simulink model "NMM_order6_multi2"  (R2023a)
settings: Solver=VariableStepAuto  StartTime=0.0  StopTime=11.0  RelTol=1e-3
undefined symbols (not defined in the file): clf
libraries: simulink x4
(part 1 of 2)
settings Model: Creator=HP  LastModifiedBy=admin

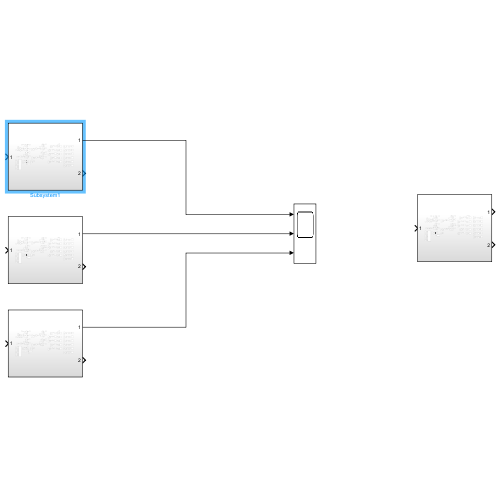
[thumbnail: Simulink's stored preview of the top-level diagram]
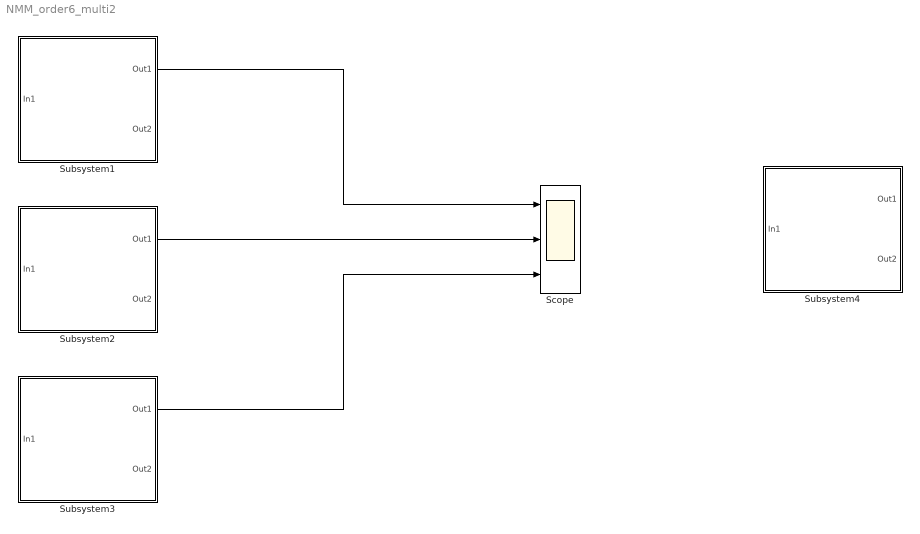
== system NMM_order6_multi2 ==
  Scope : Scope  NumInputPorts=3
  Subsystem1 : Subsystem
  Subsystem2 : Subsystem
  Subsystem3 : Subsystem
  Subsystem4 : Subsystem
  wires:
  Subsystem1/1(Out1) -> Scope/1
  Subsystem2/1(Out1) -> Scope/2
  Subsystem3/1(Out1) -> Scope/3

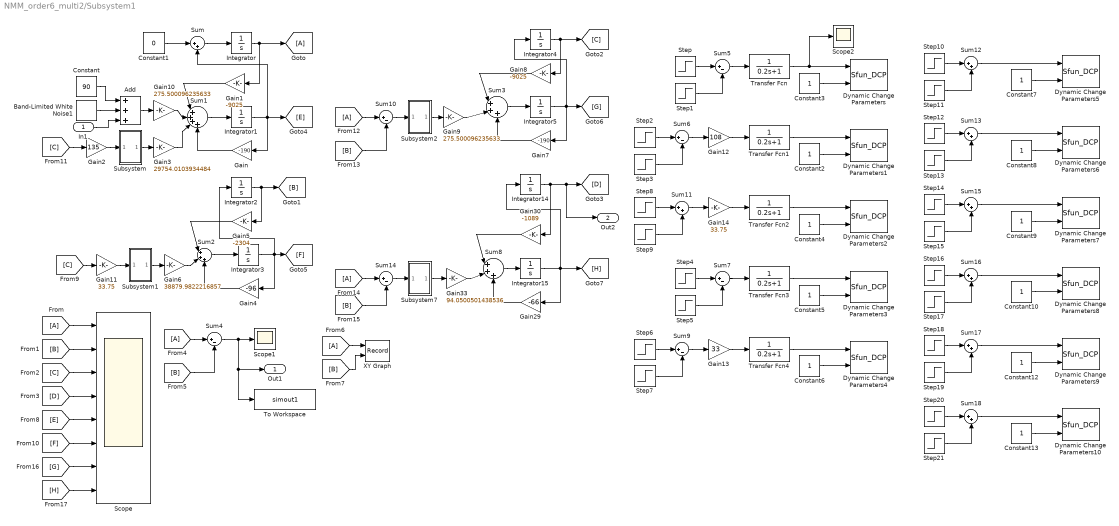
== system NMM_order6_multi2/Subsystem1 ==
  In1 : Inport
  Add : Sum  Inputs=+++
  Band-Limited White Noise1 : simulink/Sources/Band-Limited White Noise  Cov=[0.03]  Ts=0.001  seed=[23341]
  Constant : Constant  Value=90
  Constant1 : Constant  Value=0
  Constant{2..10,12..13} (11 alike) : Constant
  Dynamic Change Parameters : M-S-Function  StopFcn=close(clf)  FunctionName=Sfun_DCP  Parameters=block_name,par_name,sample_time,dimension  mask{block_name='NMM_order6_multi2/Subsystem1/Gain10', par_name='Gain', reset=off, sample_time=[0.01 0], dimension=[1 1]}
      mask help:
      | Dynamic Change Parameters : Change Block's Parameter When the Model is running
      |
      | block_name : name of the block  need to change parameter,must be string
      | par_name   : name of the parameter want to change,must be string
      | sample_time: sample time of this block
      | demension  : demension of the parameter want to change,must be [m n]
      mask Callback reset:
      | if strcmp( get_param(gcb,'reset'),'on' )
      |    fig_par_set();
      | end
      mask Callback sample_time:
      | st = get_param(gcb,'sample_time');
      | st = str2num(st);
      | if length(st)~=2
      |     msgbox('Sample Time is invalid ');
      | end
      mask Callback dimension:
      | st = get_param(gcb,'dimension');
      | st = str2num(st);
      | if length(st)~=2
      |     msgbox('Fromat of Dimension must be [m n]');
      | end
  Dynamic Change Parameters1 : M-S-Function  StopFcn=close(clf)  FunctionName=Sfun_DCP  Parameters=block_name,par_name,sample_time,dimension  mask{block_name='NMM_order6_multi2/Subsystem1/Gain3', par_name='Gain', reset=off, sample_time=[0.01 0], dimension=[1 1]}
      mask help:
      | Dynamic Change Parameters : Change Block's Parameter When the Model is running
      |
      | block_name : name of the block  need to change parameter,must be string
      | par_name   : name of the parameter want to change,must be string
      | sample_time: sample time of this block
      | demension  : demension of the parameter want to change,must be [m n]
      mask Callback reset:
      | if strcmp( get_param(gcb,'reset'),'on' )
      |    fig_par_set();
      | end
      mask Callback sample_time:
      | st = get_param(gcb,'sample_time');
      | st = str2num(st);
      | if length(st)~=2
      |     msgbox('Sample Time is invalid ');
      | end
      mask Callback dimension:
      | st = get_param(gcb,'dimension');
      | st = str2num(st);
      | if length(st)~=2
      |     msgbox('Fromat of Dimension must be [m n]');
      | end
  Dynamic Change Parameters10 : M-S-Function  StopFcn=close(clf)  FunctionName=Sfun_DCP  Parameters=block_name,par_name,sample_time,dimension  mask{block_name='NMM_order6_multi2/Subsystem1/Gain7', par_name='Gain', reset=off, sample_time=[0.01 0], dimension=[1 1]}
      mask help:
      | Dynamic Change Parameters : Change Block's Parameter When the Model is running
      |
      | block_name : name of the block  need to change parameter,must be string
      | par_name   : name of the parameter want to change,must be string
      | sample_time: sample time of this block
      | demension  : demension of the parameter want to change,must be [m n]
      mask Callback reset:
      | if strcmp( get_param(gcb,'reset'),'on' )
      |    fig_par_set();
      | end
      mask Callback sample_time:
      | st = get_param(gcb,'sample_time');
      | st = str2num(st);
      | if length(st)~=2
      |     msgbox('Sample Time is invalid ');
      | end
      mask Callback dimension:
      | st = get_param(gcb,'dimension');
      | st = str2num(st);
      | if length(st)~=2
      |     msgbox('Fromat of Dimension must be [m n]');
      | end
  Dynamic Change Parameters2 : M-S-Function  StopFcn=close(clf)  FunctionName=Sfun_DCP  Parameters=block_name,par_name,sample_time,dimension  mask{block_name='NMM_order6_multi2/Subsystem1/Gain6', par_name='Gain', reset=off, sample_time=[0.01 0], dimension=[1 1]}
      mask help:
      | Dynamic Change Parameters : Change Block's Parameter When the Model is running
      |
      | block_name : name of the block  need to change parameter,must be string
      | par_name   : name of the parameter want to change,must be string
      | sample_time: sample time of this block
      | demension  : demension of the parameter want to change,must be [m n]
      mask Callback reset:
      | if strcmp( get_param(gcb,'reset'),'on' )
      |    fig_par_set();
      | end
      mask Callback sample_time:
      | st = get_param(gcb,'sample_time');
      | st = str2num(st);
      | if length(st)~=2
      |     msgbox('Sample Time is invalid ');
      | end
      mask Callback dimension:
      | st = get_param(gcb,'dimension');
      | st = str2num(st);
      | if length(st)~=2
      |     msgbox('Fromat of Dimension must be [m n]');
      | end
  Dynamic Change Parameters3 : M-S-Function  StopFcn=close(clf)  FunctionName=Sfun_DCP  Parameters=block_name,par_name,sample_time,dimension  mask{block_name='NMM_order6_multi2/Subsystem1/Gain9', par_name='Gain', reset=off, sample_time=[0.01 0], dimension=[1 1]}
      mask help:
      | Dynamic Change Parameters : Change Block's Parameter When the Model is running
      |
      | block_name : name of the block  need to change parameter,must be string
      | par_name   : name of the parameter want to change,must be string
      | sample_time: sample time of this block
      | demension  : demension of the parameter want to change,must be [m n]
      mask Callback reset:
      | if strcmp( get_param(gcb,'reset'),'on' )
      |    fig_par_set();
      | end
      mask Callback sample_time:
      | st = get_param(gcb,'sample_time');
      | st = str2num(st);
      | if length(st)~=2
      |     msgbox('Sample Time is invalid ');
      | end
      mask Callback dimension:
      | st = get_param(gcb,'dimension');
      | st = str2num(st);
      | if length(st)~=2
      |     msgbox('Fromat of Dimension must be [m n]');
      | end
  Dynamic Change Parameters4 : M-S-Function  StopFcn=close(clf)  FunctionName=Sfun_DCP  Parameters=block_name,par_name,sample_time,dimension  mask{block_name='NMM_order6_multi2/Subsystem1/Gain33', par_name='Gain', reset=off, sample_time=[0.01 0], dimension=[1 1]}
      mask help:
      | Dynamic Change Parameters : Change Block's Parameter When the Model is running
      |
      | block_name : name of the block  need to change parameter,must be string
      | par_name   : name of the parameter want to change,must be string
      | sample_time: sample time of this block
      | demension  : demension of the parameter want to change,must be [m n]
      mask Callback reset:
      | if strcmp( get_param(gcb,'reset'),'on' )
      |    fig_par_set();
      | end
      mask Callback sample_time:
      | st = get_param(gcb,'sample_time');
      | st = str2num(st);
      | if length(st)~=2
      |     msgbox('Sample Time is invalid ');
      | end
      mask Callback dimension:
      | st = get_param(gcb,'dimension');
      | st = str2num(st);
      | if length(st)~=2
      |     msgbox('Fromat of Dimension must be [m n]');
      | end
  Dynamic Change Parameters5 : M-S-Function  StopFcn=close(clf)  FunctionName=Sfun_DCP  Parameters=block_name,par_name,sample_time,dimension  mask{block_name='NMM_order6_multi2/Subsystem1/Gain1', par_name='Gain', reset=off, sample_time=[0.01 0], dimension=[1 1]}
      mask help:
      | Dynamic Change Parameters : Change Block's Parameter When the Model is running
      |
      | block_name : name of the block  need to change parameter,must be string
      | par_name   : name of the parameter want to change,must be string
      | sample_time: sample time of this block
      | demension  : demension of the parameter want to change,must be [m n]
      mask Callback reset:
      | if strcmp( get_param(gcb,'reset'),'on' )
      |    fig_par_set();
      | end
      mask Callback sample_time:
      | st = get_param(gcb,'sample_time');
      | st = str2num(st);
      | if length(st)~=2
      |     msgbox('Sample Time is invalid ');
      | end
      mask Callback dimension:
      | st = get_param(gcb,'dimension');
      | st = str2num(st);
      | if length(st)~=2
      |     msgbox('Fromat of Dimension must be [m n]');
      | end
  Dynamic Change Parameters6 : M-S-Function  StopFcn=close(clf)  FunctionName=Sfun_DCP  Parameters=block_name,par_name,sample_time,dimension  mask{block_name='NMM_order6_multi2/Subsystem1/Gain', par_name='Gain', reset=off, sample_time=[0.01 0], dimension=[1 1]}
      mask help:
      | Dynamic Change Parameters : Change Block's Parameter When the Model is running
      |
      | block_name : name of the block  need to change parameter,must be string
      | par_name   : name of the parameter want to change,must be string
      | sample_time: sample time of this block
      | demension  : demension of the parameter want to change,must be [m n]
      mask Callback reset:
      | if strcmp( get_param(gcb,'reset'),'on' )
      |    fig_par_set();
      | end
      mask Callback sample_time:
      | st = get_param(gcb,'sample_time');
      | st = str2num(st);
      | if length(st)~=2
      |     msgbox('Sample Time is invalid ');
      | end
      mask Callback dimension:
      | st = get_param(gcb,'dimension');
      | st = str2num(st);
      | if length(st)~=2
      |     msgbox('Fromat of Dimension must be [m n]');
      | end
  Dynamic Change Parameters7 : M-S-Function  StopFcn=close(clf)  FunctionName=Sfun_DCP  Parameters=block_name,par_name,sample_time,dimension  mask{block_name='NMM_order6_multi2/Subsystem1/Gain5', par_name='Gain', reset=off, sample_time=[0.01 0], dimension=[1 1]}
      mask help:
      | Dynamic Change Parameters : Change Block's Parameter When the Model is running
      |
      | block_name : name of the block  need to change parameter,must be string
      | par_name   : name of the parameter want to change,must be string
      | sample_time: sample time of this block
      | demension  : demension of the parameter want to change,must be [m n]
      mask Callback reset:
      | if strcmp( get_param(gcb,'reset'),'on' )
      |    fig_par_set();
      | end
      mask Callback sample_time:
      | st = get_param(gcb,'sample_time');
      | st = str2num(st);
      | if length(st)~=2
      |     msgbox('Sample Time is invalid ');
      | end
      mask Callback dimension:
      | st = get_param(gcb,'dimension');
      | st = str2num(st);
      | if length(st)~=2
      |     msgbox('Fromat of Dimension must be [m n]');
      | end
  Dynamic Change Parameters8 : M-S-Function  StopFcn=close(clf)  FunctionName=Sfun_DCP  Parameters=block_name,par_name,sample_time,dimension  mask{block_name='NMM_order6_multi2/Subsystem1/Gain4', par_name='Gain', reset=off, sample_time=[0.01 0], dimension=[1 1]}
      mask help:
      | Dynamic Change Parameters : Change Block's Parameter When the Model is running
      |
      | block_name : name of the block  need to change parameter,must be string
      | par_name   : name of the parameter want to change,must be string
      | sample_time: sample time of this block
      | demension  : demension of the parameter want to change,must be [m n]
      mask Callback reset:
      | if strcmp( get_param(gcb,'reset'),'on' )
      |    fig_par_set();
      | end
      mask Callback sample_time:
      | st = get_param(gcb,'sample_time');
      | st = str2num(st);
      | if length(st)~=2
      |     msgbox('Sample Time is invalid ');
      | end
      mask Callback dimension:
      | st = get_param(gcb,'dimension');
      | st = str2num(st);
      | if length(st)~=2
      |     msgbox('Fromat of Dimension must be [m n]');
      | end
  Dynamic Change Parameters9 : M-S-Function  StopFcn=close(clf)  FunctionName=Sfun_DCP  Parameters=block_name,par_name,sample_time,dimension  mask{block_name='NMM_order6_multi2/Subsystem1/Gain8', par_name='Gain', reset=off, sample_time=[0.01 0], dimension=[1 1]}
      mask help:
      | Dynamic Change Parameters : Change Block's Parameter When the Model is running
      |
      | block_name : name of the block  need to change parameter,must be string
      | par_name   : name of the parameter want to change,must be string
      | sample_time: sample time of this block
      | demension  : demension of the parameter want to change,must be [m n]
      mask Callback reset:
      | if strcmp( get_param(gcb,'reset'),'on' )
      |    fig_par_set();
      | end
      mask Callback sample_time:
      | st = get_param(gcb,'sample_time');
      | st = str2num(st);
      | if length(st)~=2
      |     msgbox('Sample Time is invalid ');
      | end
      mask Callback dimension:
      | st = get_param(gcb,'dimension');
      | st = str2num(st);
      | if length(st)~=2
      |     msgbox('Fromat of Dimension must be [m n]');
      | end
  From{,4,6,12,14} (5 alike) : From
  Gain : Gain  Gain=-190
  Gain1 : Gain  Gain=-9025
  Gain10 : Gain  Gain=275.500096235633
  Gain11 : Gain  Gain=33.75
  Gain12 : Gain  Gain=108
  Gain13 : Gain  Gain=33
  Gain14 : Gain  Gain=33.75
  Gain2 : Gain  Gain=135
  Gain29 : Gain  Gain=-66
  Gain3 : Gain  Gain=29754.0103934484
  Gain30 : Gain  Gain=-1089
  Gain33 : Gain  Gain=94.0500501438536
  Gain4 : Gain  Gain=-96
  Gain5 : Gain  Gain=-2304
  Gain6 : Gain  Gain=38879.9822216857
  Gain7 : Gain  Gain=-190
  Gain8 : Gain  Gain=-9025
  Gain9 : Gain  Gain=275.500096235633
  Goto : Goto
  Integrator{,1..5,14..15} (8 alike) : Integrator
  Scope : Scope  NumInputPorts=8
  Scope1 : Scope
  Scope2 : Scope
  Step : Step  Time=5.8  Before=2.35*100  After=3.00*95  SampleTime=0
  Step1 : Step  Time=8.7  After=9.5  SampleTime=0
  Step10 : Step  Time=5.8  Before=-10000  After=-9025  SampleTime=0
  Step{11,13,15,17,19,21} (6 alike) : Step  Time=8.7  After=0  SampleTime=0
  Step12 : Step  Time=5.8  Before=-200  After=-190  SampleTime=0
  Step14 : Step  Time=5.8  Before=-2500  After=-2304  SampleTime=0
  Step16 : Step  Time=5.8  Before=-100  After=-96  SampleTime=0
  Step18 : Step  Time=5.8  Before=-10000  After=-9025  SampleTime=0
  Step2 : Step  Time=5.8  Before=2.35*100  After=3.00*95  SampleTime=0
  Step20 : Step  Time=5.8  Before=-200  After=-190  SampleTime=0
  Step3 : Step  Time=8.7  After=9.5  SampleTime=0
  Step4 : Step  Time=5.8  Before=2.35*100  After=3.00*95  SampleTime=0
  Step5 : Step  Time=8.7  After=9.5  SampleTime=0
  Step6 : Step  Time=5.8  Before=2.35  After=3.00  SampleTime=0
  Step7 : Step  Time=8.7  After=0.15  SampleTime=0
  Step8 : Step  Time=20  Before=22*50  After=22*50  SampleTime=0
  Step9 : Step  Time=8.7  After=52  SampleTime=0
  Subsystem : Subsystem
  Subsystem1 : Subsystem
  Subsystem2 : Subsystem
  Subsystem7 : Subsystem
  Sum{,11..13,15..18} (8 alike) : Sum  Inputs=|++
  Sum1 : Sum  Inputs=|++++
  Sum{4..7,9..10,14} (7 alike) : Sum  Inputs=|+-
  Sum2 : Sum  Inputs=|+++
  Sum3 : Sum  Inputs=|+++
  Sum8 : Sum  Inputs=|+++
  To Workspace : ToWorkspace  VariableName=simout1  SaveFormat=Timeseries  SampleTime=-1
  Transfer Fcn{,1..4} (5 alike) : TransferFcn  Denominator=[0.2 1]
  XY Graph : Record  FileSettingsInternal="{\"entries\":[{\"content\":{\"excelSettings\":{\"content\":{},\"type\":\"Streamout.ExcelSettings\"}},\"type\":\"Streamout.FileSettingStorage\",\"uuid\":\"\"}],\"packageUris\":[\"http:\\/\\/schema.mathworks.com\\/mf0\\/streamout_blocks\\/R2020a\"],\"version\":\"1.0\"}"  Layout=[1 1]  SignalsInternal="{\"entries\":[{\"content\":{\"signals\":[{\"content\":{\"blockPath\":[],\"dimensions\":[1],\"domain\":\"\",\"lineColor\":\"#77ac30\",\"port\":1,\"sid\":[\"\"],\"signalID\":93784,\"signalName\":\"From6\"},\"type\":\"RecordBlkView.Signal\",\"uuid\":\"\"},{\"content\":{\"blockPath\":[],\"dimensions\":[1],\"domain\":\"\",\"lineColor\":\"#4dbeee\",\"port\":2,\"sid\":[\"\"],\"signalID\":93788,\"signalName\":\"From7\"},\"type\":\"RecordBlkView.Signal\",\"uuid\":\"\"}]},\"type\":\"RecordBlkView.InputSignals\",\"uuid\":\"\"}],\"packageUris\":[\"http:\\/\\/schema.mathworks.com\\/mf0\\/streamout_blocks\\/R2020a\"],\"version\":\"1.0\"}"  VisualizationBindings="{\"xyplotplugin\":{\"info\":[{\"series\":[],\"subplotID\":1}]}}"  CompatibilityTag=XY
  Out1 : Outport
  Out2 : Outport  Port=2
  wires:
  Sum4/1 -> To Workspace/1, Out1/1, Scope1/1
  [C] -> Scope/3
  Gain1/1 -> Sum1/1
  Sum1/1 -> Integrator1/1
  Subsystem2/1(Out2) -> Gain9/1
  [B] -> Sum10/2
  [G] -> Scope/7
  Subsystem/1(Out2) -> Gain3/1
  Gain4/1 -> Sum2/3
  Gain9/1 -> Sum3/2
  [D] -> Scope/4
  Integrator4/1 -> [C], Gain8/1
  Sum/1 -> Integrator/1
  Gain3/1 -> Sum1/3
  Gain30/1 -> Sum8/1
  From/1 -> Scope/1
  Constant/1 -> Add/1
  [B] -> Scope/2
  From6/1 -> XY Graph/1
  Add/1 -> Gain10/1
  Integrator5/1 -> [G], Gain7/1, Integrator4/1
  Gain/1 -> Sum1/4
  Integrator2/1 -> [B], Gain5/1
  [H] -> Scope/8
  [B] -> Sum14/2
  Integrator1/1 -> [E], Sum/2, Gain/1
  Integrator/1 -> Goto/1, Gain1/1
  Gain6/1 -> Sum2/2
  Sum8/1 -> Integrator15/1
  Integrator3/1 -> [F], Gain4/1, Integrator2/1
  Gain5/1 -> Sum2/1
  Gain8/1 -> Sum3/1
  Integrator14/1 -> Out2/1, [D], Gain30/1
  Integrator15/1 -> [H], Gain29/1, Integrator14/1
  Subsystem1/1(Out2) -> Gain6/1
  From14/1 -> Sum14/1
  Gain2/1 -> Subsystem/1(In1)
  Sum14/1 -> Subsystem7/1(In1)
  Sum10/1 -> Subsystem2/1(In1)
  Gain33/1 -> Sum8/2
  Gain29/1 -> Sum8/3
  [C] -> Gain11/1
  Subsystem7/1(Out2) -> Gain33/1
  Gain7/1 -> Sum3/3
  [B] -> Sum4/2
  From4/1 -> Sum4/1
  Band-Limited White Noise1/1 -> Add/2
  In1/1 -> Add/3
  Sum3/1 -> Integrator5/1
  Constant1/1 -> Sum/1
  Gain11/1 -> Subsystem1/1(In1)
  [E] -> Scope/5
  [C] -> Gain2/1
  Sum2/1 -> Integrator3/1
  [F] -> Scope/6
  Gain10/1 -> Sum1/2
  From12/1 -> Sum10/1
  [B] -> XY Graph/2
  Constant3/1 -> Dynamic Change Parameters/2
  Constant2/1 -> Dynamic Change Parameters1/2
  Constant5/1 -> Dynamic Change Parameters3/2
  Constant6/1 -> Dynamic Change Parameters4/2
  Step/1 -> Sum5/1
  Step1/1 -> Sum5/2
  Step3/1 -> Sum6/2
  Step2/1 -> Sum6/1
  Sum6/1 -> Gain12/1
  Step5/1 -> Sum7/2
  Step4/1 -> Sum7/1
  Step7/1 -> Sum9/2
  Step6/1 -> Sum9/1
  Sum9/1 -> Gain13/1
  Step9/1 -> Sum11/2
  Step8/1 -> Sum11/1
  Sum11/1 -> Gain14/1
  Constant4/1 -> Dynamic Change Parameters2/2
  Sum5/1 -> Transfer Fcn/1
  Transfer Fcn/1 -> Scope2/1, Dynamic Change Parameters/1
  Transfer Fcn1/1 -> Dynamic Change Parameters1/1
  Gain12/1 -> Transfer Fcn1/1
  Gain14/1 -> Transfer Fcn2/1
  Transfer Fcn2/1 -> Dynamic Change Parameters2/1
  Sum7/1 -> Transfer Fcn3/1
  Transfer Fcn3/1 -> Dynamic Change Parameters3/1
  Gain13/1 -> Transfer Fcn4/1
  Transfer Fcn4/1 -> Dynamic Change Parameters4/1
  Step11/1 -> Sum12/2
  Constant7/1 -> Dynamic Change Parameters5/2
  Step10/1 -> Sum12/1
  Step13/1 -> Sum13/2
  Constant8/1 -> Dynamic Change Parameters6/2
  Step12/1 -> Sum13/1
  Step16/1 -> Sum16/1
  Constant10/1 -> Dynamic Change Parameters8/2
  Step17/1 -> Sum16/2
  Constant9/1 -> Dynamic Change Parameters7/2
  Step15/1 -> Sum15/2
  Step14/1 -> Sum15/1
  Constant13/1 -> Dynamic Change Parameters10/2
  Step21/1 -> Sum18/2
  Step19/1 -> Sum17/2
  Constant12/1 -> Dynamic Change Parameters9/2
  Step20/1 -> Sum18/1
  Step18/1 -> Sum17/1
  Sum12/1 -> Dynamic Change Parameters5/1
  Sum13/1 -> Dynamic Change Parameters6/1
  Sum15/1 -> Dynamic Change Parameters7/1
  Sum16/1 -> Dynamic Change Parameters8/1
  Sum17/1 -> Dynamic Change Parameters9/1
  Sum18/1 -> Dynamic Change Parameters10/1

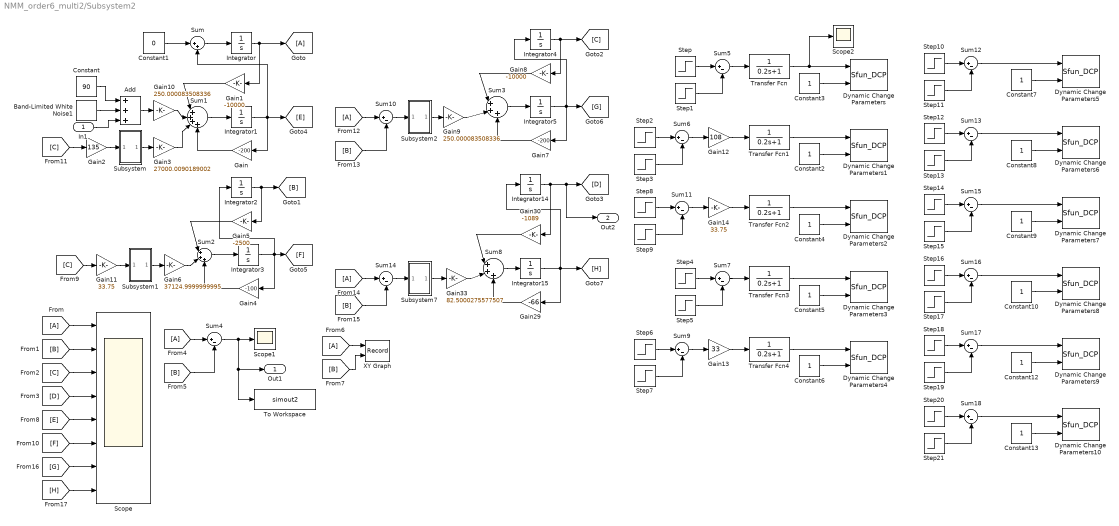
== system NMM_order6_multi2/Subsystem2 ==
  In1 : Inport
  Add : Sum  Inputs=+++
  Band-Limited White Noise1 : simulink/Sources/Band-Limited White Noise  Cov=[0.01]  Ts=0.001  seed=[35471]
  Constant : Constant  Value=90
  Constant1 : Constant  Value=0
  Constant{2..10,12..13} (11 alike) : Constant
  Dynamic Change Parameters : M-S-Function  StopFcn=close(clf)  FunctionName=Sfun_DCP  Parameters=block_name,par_name,sample_time,dimension  mask{block_name='NMM_order6_multi2/Subsystem2/Gain10', par_name='Gain', reset=off, sample_time=[0.01 0], dimension=[1 1]}
      mask help:
      | Dynamic Change Parameters : Change Block's Parameter When the Model is running
      |
      | block_name : name of the block  need to change parameter,must be string
      | par_name   : name of the parameter want to change,must be string
      | sample_time: sample time of this block
      | demension  : demension of the parameter want to change,must be [m n]
      mask Callback reset:
      | if strcmp( get_param(gcb,'reset'),'on' )
      |    fig_par_set();
      | end
      mask Callback sample_time:
      | st = get_param(gcb,'sample_time');
      | st = str2num(st);
      | if length(st)~=2
      |     msgbox('Sample Time is invalid ');
      | end
      mask Callback dimension:
      | st = get_param(gcb,'dimension');
      | st = str2num(st);
      | if length(st)~=2
      |     msgbox('Fromat of Dimension must be [m n]');
      | end
  Dynamic Change Parameters1 : M-S-Function  StopFcn=close(clf)  FunctionName=Sfun_DCP  Parameters=block_name,par_name,sample_time,dimension  mask{block_name='NMM_order6_multi2/Subsystem2/Gain3', par_name='Gain', reset=off, sample_time=[0.01 0], dimension=[1 1]}
      mask help:
      | Dynamic Change Parameters : Change Block's Parameter When the Model is running
      |
      | block_name : name of the block  need to change parameter,must be string
      | par_name   : name of the parameter want to change,must be string
      | sample_time: sample time of this block
      | demension  : demension of the parameter want to change,must be [m n]
      mask Callback reset:
      | if strcmp( get_param(gcb,'reset'),'on' )
      |    fig_par_set();
      | end
      mask Callback sample_time:
      | st = get_param(gcb,'sample_time');
      | st = str2num(st);
      | if length(st)~=2
      |     msgbox('Sample Time is invalid ');
      | end
      mask Callback dimension:
      | st = get_param(gcb,'dimension');
      | st = str2num(st);
      | if length(st)~=2
      |     msgbox('Fromat of Dimension must be [m n]');
      | end
  Dynamic Change Parameters10 : M-S-Function  StopFcn=close(clf)  FunctionName=Sfun_DCP  Parameters=block_name,par_name,sample_time,dimension  mask{block_name='NMM_order6_multi2/Subsystem2/Gain7', par_name='Gain', reset=off, sample_time=[0.01 0], dimension=[1 1]}
      mask help:
      | Dynamic Change Parameters : Change Block's Parameter When the Model is running
      |
      | block_name : name of the block  need to change parameter,must be string
      | par_name   : name of the parameter want to change,must be string
      | sample_time: sample time of this block
      | demension  : demension of the parameter want to change,must be [m n]
      mask Callback reset:
      | if strcmp( get_param(gcb,'reset'),'on' )
      |    fig_par_set();
      | end
      mask Callback sample_time:
      | st = get_param(gcb,'sample_time');
      | st = str2num(st);
      | if length(st)~=2
      |     msgbox('Sample Time is invalid ');
      | end
      mask Callback dimension:
      | st = get_param(gcb,'dimension');
      | st = str2num(st);
      | if length(st)~=2
      |     msgbox('Fromat of Dimension must be [m n]');
      | end
  Dynamic Change Parameters2 : M-S-Function  StopFcn=close(clf)  FunctionName=Sfun_DCP  Parameters=block_name,par_name,sample_time,dimension  mask{block_name='NMM_order6_multi2/Subsystem2/Gain6', par_name='Gain', reset=off, sample_time=[0.01 0], dimension=[1 1]}
      mask help:
      | Dynamic Change Parameters : Change Block's Parameter When the Model is running
      |
      | block_name : name of the block  need to change parameter,must be string
      | par_name   : name of the parameter want to change,must be string
      | sample_time: sample time of this block
      | demension  : demension of the parameter want to change,must be [m n]
      mask Callback reset:
      | if strcmp( get_param(gcb,'reset'),'on' )
      |    fig_par_set();
      | end
      mask Callback sample_time:
      | st = get_param(gcb,'sample_time');
      | st = str2num(st);
      | if length(st)~=2
      |     msgbox('Sample Time is invalid ');
      | end
      mask Callback dimension:
      | st = get_param(gcb,'dimension');
      | st = str2num(st);
      | if length(st)~=2
      |     msgbox('Fromat of Dimension must be [m n]');
      | end
  Dynamic Change Parameters3 : M-S-Function  StopFcn=close(clf)  FunctionName=Sfun_DCP  Parameters=block_name,par_name,sample_time,dimension  mask{block_name='NMM_order6_multi2/Subsystem2/Gain9', par_name='Gain', reset=off, sample_time=[0.01 0], dimension=[1 1]}
      mask help:
      | Dynamic Change Parameters : Change Block's Parameter When the Model is running
      |
      | block_name : name of the block  need to change parameter,must be string
      | par_name   : name of the parameter want to change,must be string
      | sample_time: sample time of this block
      | demension  : demension of the parameter want to change,must be [m n]
      mask Callback reset:
      | if strcmp( get_param(gcb,'reset'),'on' )
      |    fig_par_set();
      | end
      mask Callback sample_time:
      | st = get_param(gcb,'sample_time');
      | st = str2num(st);
      | if length(st)~=2
      |     msgbox('Sample Time is invalid ');
      | end
      mask Callback dimension:
      | st = get_param(gcb,'dimension');
      | st = str2num(st);
      | if length(st)~=2
      |     msgbox('Fromat of Dimension must be [m n]');
      | end
  Dynamic Change Parameters4 : M-S-Function  StopFcn=close(clf)  FunctionName=Sfun_DCP  Parameters=block_name,par_name,sample_time,dimension  mask{block_name='NMM_order6_multi2/Subsystem2/Gain33', par_name='Gain', reset=off, sample_time=[0.01 0], dimension=[1 1]}
      mask help:
      | Dynamic Change Parameters : Change Block's Parameter When the Model is running
      |
      | block_name : name of the block  need to change parameter,must be string
      | par_name   : name of the parameter want to change,must be string
      | sample_time: sample time of this block
      | demension  : demension of the parameter want to change,must be [m n]
      mask Callback reset:
      | if strcmp( get_param(gcb,'reset'),'on' )
      |    fig_par_set();
      | end
      mask Callback sample_time:
      | st = get_param(gcb,'sample_time');
      | st = str2num(st);
      | if length(st)~=2
      |     msgbox('Sample Time is invalid ');
      | end
      mask Callback dimension:
      | st = get_param(gcb,'dimension');
      | st = str2num(st);
      | if length(st)~=2
      |     msgbox('Fromat of Dimension must be [m n]');
      | end
  Dynamic Change Parameters5 : M-S-Function  StopFcn=close(clf)  FunctionName=Sfun_DCP  Parameters=block_name,par_name,sample_time,dimension  mask{block_name='NMM_order6_multi2/Subsystem2/Gain1', par_name='Gain', reset=off, sample_time=[0.01 0], dimension=[1 1]}
      mask help:
      | Dynamic Change Parameters : Change Block's Parameter When the Model is running
      |
      | block_name : name of the block  need to change parameter,must be string
      | par_name   : name of the parameter want to change,must be string
      | sample_time: sample time of this block
      | demension  : demension of the parameter want to change,must be [m n]
      mask Callback reset:
      | if strcmp( get_param(gcb,'reset'),'on' )
      |    fig_par_set();
      | end
      mask Callback sample_time:
      | st = get_param(gcb,'sample_time');
      | st = str2num(st);
      | if length(st)~=2
      |     msgbox('Sample Time is invalid ');
      | end
      mask Callback dimension:
      | st = get_param(gcb,'dimension');
      | st = str2num(st);
      | if length(st)~=2
      |     msgbox('Fromat of Dimension must be [m n]');
      | end
  Dynamic Change Parameters6 : M-S-Function  StopFcn=close(clf)  FunctionName=Sfun_DCP  Parameters=block_name,par_name,sample_time,dimension  mask{block_name='NMM_order6_multi2/Subsystem2/Gain', par_name='Gain', reset=off, sample_time=[0.01 0], dimension=[1 1]}
      mask help:
      | Dynamic Change Parameters : Change Block's Parameter When the Model is running
      |
      | block_name : name of the block  need to change parameter,must be string
      | par_name   : name of the parameter want to change,must be string
      | sample_time: sample time of this block
      | demension  : demension of the parameter want to change,must be [m n]
      mask Callback reset:
      | if strcmp( get_param(gcb,'reset'),'on' )
      |    fig_par_set();
      | end
      mask Callback sample_time:
      | st = get_param(gcb,'sample_time');
      | st = str2num(st);
      | if length(st)~=2
      |     msgbox('Sample Time is invalid ');
      | end
      mask Callback dimension:
      | st = get_param(gcb,'dimension');
      | st = str2num(st);
      | if length(st)~=2
      |     msgbox('Fromat of Dimension must be [m n]');
      | end
  Dynamic Change Parameters7 : M-S-Function  StopFcn=close(clf)  FunctionName=Sfun_DCP  Parameters=block_name,par_name,sample_time,dimension  mask{block_name='NMM_order6_multi2/Subsystem2/Gain5', par_name='Gain', reset=off, sample_time=[0.01 0], dimension=[1 1]}
      mask help:
      | Dynamic Change Parameters : Change Block's Parameter When the Model is running
      |
      | block_name : name of the block  need to change parameter,must be string
      | par_name   : name of the parameter want to change,must be string
      | sample_time: sample time of this block
      | demension  : demension of the parameter want to change,must be [m n]
      mask Callback reset:
      | if strcmp( get_param(gcb,'reset'),'on' )
      |    fig_par_set();
      | end
      mask Callback sample_time:
      | st = get_param(gcb,'sample_time');
      | st = str2num(st);
      | if length(st)~=2
      |     msgbox('Sample Time is invalid ');
      | end
      mask Callback dimension:
      | st = get_param(gcb,'dimension');
      | st = str2num(st);
      | if length(st)~=2
      |     msgbox('Fromat of Dimension must be [m n]');
      | end
  Dynamic Change Parameters8 : M-S-Function  StopFcn=close(clf)  FunctionName=Sfun_DCP  Parameters=block_name,par_name,sample_time,dimension  mask{block_name='NMM_order6_multi2/Subsystem2/Gain4', par_name='Gain', reset=off, sample_time=[0.01 0], dimension=[1 1]}
      mask help:
      | Dynamic Change Parameters : Change Block's Parameter When the Model is running
      |
      | block_name : name of the block  need to change parameter,must be string
      | par_name   : name of the parameter want to change,must be string
      | sample_time: sample time of this block
      | demension  : demension of the parameter want to change,must be [m n]
      mask Callback reset:
      | if strcmp( get_param(gcb,'reset'),'on' )
      |    fig_par_set();
      | end
      mask Callback sample_time:
      | st = get_param(gcb,'sample_time');
      | st = str2num(st);
      | if length(st)~=2
      |     msgbox('Sample Time is invalid ');
      | end
      mask Callback dimension:
      | st = get_param(gcb,'dimension');
      | st = str2num(st);
      | if length(st)~=2
      |     msgbox('Fromat of Dimension must be [m n]');
      | end
  Dynamic Change Parameters9 : M-S-Function  StopFcn=close(clf)  FunctionName=Sfun_DCP  Parameters=block_name,par_name,sample_time,dimension  mask{block_name='NMM_order6_multi2/Subsystem2/Gain8', par_name='Gain', reset=off, sample_time=[0.01 0], dimension=[1 1]}
      mask help:
      | Dynamic Change Parameters : Change Block's Parameter When the Model is running
      |
      | block_name : name of the block  need to change parameter,must be string
      | par_name   : name of the parameter want to change,must be string
      | sample_time: sample time of this block
      | demension  : demension of the parameter want to change,must be [m n]
      mask Callback reset:
      | if strcmp( get_param(gcb,'reset'),'on' )
      |    fig_par_set();
      | end
      mask Callback sample_time:
      | st = get_param(gcb,'sample_time');
      | st = str2num(st);
      | if length(st)~=2
      |     msgbox('Sample Time is invalid ');
      | end
      mask Callback dimension:
      | st = get_param(gcb,'dimension');
      | st = str2num(st);
      | if length(st)~=2
      |     msgbox('Fromat of Dimension must be [m n]');
      | end
  From{,4,6,12,14} (5 alike) : From
  Gain : Gain  Gain=-200
  Gain1 : Gain  Gain=-10000
  Gain10 : Gain  Gain=250.000083508336
  Gain11 : Gain  Gain=33.75
  Gain12 : Gain  Gain=108
  Gain13 : Gain  Gain=33
  Gain14 : Gain  Gain=33.75
  Gain2 : Gain  Gain=135
  Gain29 : Gain  Gain=-66
  Gain3 : Gain  Gain=27000.0090189002
  Gain30 : Gain  Gain=-1089
  Gain33 : Gain  Gain=82.5000275577507
  Gain4 : Gain  Gain=-100
  Gain5 : Gain  Gain=-2500
  Gain6 : Gain  Gain=37124.9999999995
  Gain7 : Gain  Gain=-200
  Gain8 : Gain  Gain=-10000
  Gain9 : Gain  Gain=250.000083508336
  Goto : Goto
  Integrator{,1..5,14..15} (8 alike) : Integrator
  Scope : Scope  NumInputPorts=8
  Scope1 : Scope
  Scope2 : Scope
  Step : Step  Time=5.9  Before=2.35*100  After=2.55*100  SampleTime=0
  Step1 : Step  Time=8.8  After=0.05*100  SampleTime=0
  Step10 : Step  Time=5.8  Before=-10000  After=-10000  SampleTime=0
  Step{11,13,15,17,19,21} (6 alike) : Step  Time=8.8  After=0  SampleTime=0
  Step12 : Step  Time=5.8  Before=-200  After=-200  SampleTime=0
  Step14 : Step  Time=5.8  Before=-2500  After=-2500  SampleTime=0
  Step16 : Step  Time=5.8  Before=-100  After=-100  SampleTime=0
  Step18 : Step  Time=5.8  Before=-10000  After=-10000  SampleTime=0
  Step2 : Step  Time=5.9  Before=2.35*100  After=2.55*100  SampleTime=0
  Step20 : Step  Time=5.8  Before=-200  After=-200  SampleTime=0
  Step3 : Step  Time=8.8  After=0.05*100  SampleTime=0
  Step4 : Step  Time=5.9  Before=2.35*100  After=2.55*100  SampleTime=0
  Step5 : Step  Time=8.8  After=0.05*100  SampleTime=0
  Step6 : Step  Time=5.9  Before=2.35  After=2.55  SampleTime=0
  Step7 : Step  Time=8.8  After=0.05  SampleTime=0
  Step8 : Step  Time=20  Before=22*50  After=22*50  SampleTime=0
  Step9 : Step  Time=20  After=22*50  SampleTime=0
  Subsystem : Subsystem
  Subsystem1 : Subsystem
  Subsystem2 : Subsystem
  Subsystem7 : Subsystem
  Sum : Sum  Inputs=|++
  Sum1 : Sum  Inputs=|++++
  Sum{4..7,9..18} (14 alike) : Sum  Inputs=|+-
  Sum2 : Sum  Inputs=|+++
  Sum3 : Sum  Inputs=|+++
  Sum8 : Sum  Inputs=|+++
  To Workspace : ToWorkspace  VariableName=simout2  SaveFormat=Timeseries  SampleTime=-1
  Transfer Fcn{,1..4} (5 alike) : TransferFcn  Denominator=[0.2 1]
  XY Graph : Record  FileSettingsInternal="{\"entries\":[{\"content\":{\"excelSettings\":{\"content\":{},\"type\":\"Streamout.ExcelSettings\"}},\"type\":\"Streamout.FileSettingStorage\",\"uuid\":\"\"}],\"packageUris\":[\"http:\\/\\/schema.mathworks.com\\/mf0\\/streamout_blocks\\/R2020a\"],\"version\":\"1.0\"}"  Layout=[1 1]  SignalsInternal="{\"entries\":[{\"content\":{\"signals\":[{\"content\":{\"blockPath\":[],\"dimensions\":[1],\"domain\":\"\",\"lineColor\":\"#139fff\",\"port\":1,\"sid\":[\"\"],\"signalID\":93796,\"signalName\":\"From6\"},\"type\":\"RecordBlkView.Signal\",\"uuid\":\"\"},{\"content\":{\"blockPath\":[],\"dimensions\":[1],\"domain\":\"\",\"lineColor\":\"#ff6929\",\"port\":2,\"sid\":[\"\"],\"signalID\":93800,\"signalName\":\"From7\"},\"type\":\"RecordBlkView.Signal\",\"uuid\":\"\"}]},\"type\":\"RecordBlkView.InputSignals\",\"uuid\":\"\"}],\"packageUris\":[\"http:\\/\\/schema.mathworks.com\\/mf0\\/streamout_blocks\\/R2020a\"],\"version\":\"1.0\"}"  VisualizationBindings="{\"xyplotplugin\":{\"info\":[{\"series\":[],\"subplotID\":1}]}}"  CompatibilityTag=XY
  Out1 : Outport
  Out2 : Outport  Port=2
  wires:
  Sum4/1 -> To Workspace/1, Out1/1, Scope1/1
  [C] -> Scope/3
  Gain1/1 -> Sum1/1
  Sum1/1 -> Integrator1/1
  Subsystem2/1(Out2) -> Gain9/1
  [B] -> Sum10/2
  [G] -> Scope/7
  Subsystem/1(Out2) -> Gain3/1
  Gain4/1 -> Sum2/3
  Gain9/1 -> Sum3/2
  [D] -> Scope/4
  Integrator4/1 -> [C], Gain8/1
  Sum/1 -> Integrator/1
  Gain3/1 -> Sum1/3
  Gain30/1 -> Sum8/1
  From/1 -> Scope/1
  Constant/1 -> Add/1
  [B] -> Scope/2
  From6/1 -> XY Graph/1
  Add/1 -> Gain10/1
  Integrator5/1 -> [G], Gain7/1, Integrator4/1
  Gain/1 -> Sum1/4
  Integrator2/1 -> [B], Gain5/1
  [H] -> Scope/8
  [B] -> Sum14/2
  Integrator1/1 -> [E], Sum/2, Gain/1
  Integrator/1 -> Goto/1, Gain1/1
  Gain6/1 -> Sum2/2
  Sum8/1 -> Integrator15/1
  Integrator3/1 -> [F], Gain4/1, Integrator2/1
  Gain5/1 -> Sum2/1
  Gain8/1 -> Sum3/1
  Integrator14/1 -> Out2/1, [D], Gain30/1
  Integrator15/1 -> [H], Gain29/1, Integrator14/1
  Subsystem1/1(Out2) -> Gain6/1
  From14/1 -> Sum14/1
  Gain2/1 -> Subsystem/1(In1)
  Sum14/1 -> Subsystem7/1(In1)
  Sum10/1 -> Subsystem2/1(In1)
  Gain33/1 -> Sum8/2
  Gain29/1 -> Sum8/3
  [C] -> Gain11/1
  Subsystem7/1(Out2) -> Gain33/1
  Gain7/1 -> Sum3/3
  [B] -> Sum4/2
  From4/1 -> Sum4/1
  Band-Limited White Noise1/1 -> Add/2
  In1/1 -> Add/3
  Sum3/1 -> Integrator5/1
  Constant1/1 -> Sum/1
  Gain11/1 -> Subsystem1/1(In1)
  [E] -> Scope/5
  [C] -> Gain2/1
  Sum2/1 -> Integrator3/1
  [F] -> Scope/6
  Gain10/1 -> Sum1/2
  From12/1 -> Sum10/1
  [B] -> XY Graph/2
  Constant3/1 -> Dynamic Change Parameters/2
  Constant2/1 -> Dynamic Change Parameters1/2
  Constant5/1 -> Dynamic Change Parameters3/2
  Constant6/1 -> Dynamic Change Parameters4/2
  Step/1 -> Sum5/1
  Step1/1 -> Sum5/2
  Step3/1 -> Sum6/2
  Step2/1 -> Sum6/1
  Sum6/1 -> Gain12/1
  Step5/1 -> Sum7/2
  Step4/1 -> Sum7/1
  Step7/1 -> Sum9/2
  Step6/1 -> Sum9/1
  Sum9/1 -> Gain13/1
  Step9/1 -> Sum11/2
  Step8/1 -> Sum11/1
  Sum11/1 -> Gain14/1
  Constant4/1 -> Dynamic Change Parameters2/2
  Sum5/1 -> Transfer Fcn/1
  Transfer Fcn/1 -> Scope2/1, Dynamic Change Parameters/1
  Transfer Fcn1/1 -> Dynamic Change Parameters1/1
  Gain12/1 -> Transfer Fcn1/1
  Gain14/1 -> Transfer Fcn2/1
  Transfer Fcn2/1 -> Dynamic Change Parameters2/1
  Sum7/1 -> Transfer Fcn3/1
  Transfer Fcn3/1 -> Dynamic Change Parameters3/1
  Gain13/1 -> Transfer Fcn4/1
  Transfer Fcn4/1 -> Dynamic Change Parameters4/1
  Sum12/1 -> Dynamic Change Parameters5/1
  Step11/1 -> Sum12/2
  Constant7/1 -> Dynamic Change Parameters5/2
  Step10/1 -> Sum12/1
  Sum13/1 -> Dynamic Change Parameters6/1
  Step13/1 -> Sum13/2
  Constant8/1 -> Dynamic Change Parameters6/2
  Step12/1 -> Sum13/1
  Step16/1 -> Sum16/1
  Constant10/1 -> Dynamic Change Parameters8/2
  Sum16/1 -> Dynamic Change Parameters8/1
  Step17/1 -> Sum16/2
  Constant9/1 -> Dynamic Change Parameters7/2
  Step15/1 -> Sum15/2
  Step14/1 -> Sum15/1
  Sum15/1 -> Dynamic Change Parameters7/1
  Constant13/1 -> Dynamic Change Parameters10/2
  Sum18/1 -> Dynamic Change Parameters10/1
  Step21/1 -> Sum18/2
  Step19/1 -> Sum17/2
  Constant12/1 -> Dynamic Change Parameters9/2
  Sum17/1 -> Dynamic Change Parameters9/1
  Step20/1 -> Sum18/1
  Step18/1 -> Sum17/1
